simulink model "rayTrace_th"  (R2018b)
settings: Solver=VariableStepAuto  StartTime=0.0  StopTime=0  RelTol=1e-3
libraries: rayTrace_ul x4
settings Model: Creator=asiddiq2  LastModifiedBy=asiddiq2

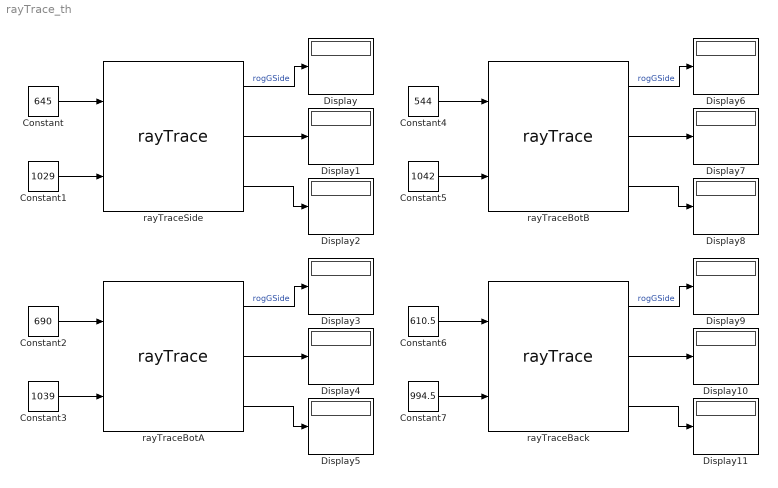
== system rayTrace_th ==
  Constant : Constant  Value=645
  Constant1 : Constant  Value=1029
  Constant2 : Constant  Value=690
  Constant3 : Constant  Value=1039
  Constant4 : Constant  Value=544
  Constant5 : Constant  Value=1042
  Constant6 : Constant  Value=610.5
  Constant7 : Constant  Value=994.5
  Display{,1..11} (12 alike) : Display
  rayTraceBack : rayTrace_ul/rayTrace  camPosVec_cm=params.prscpeCamPosVec_cm.Value  camEulAngles_deg=params.prscpeCamEulAng_deg.Value  dist2Glass_cm=params.prscpeDistancetoGlass_cm.Value  indOfRefVec=params.indexOfRefractionAGW.Value  glassPlane=3  glassThickness_cm=(3/16)*2.54  imageDimsVec_px=params.sideImageSize_px.Value  camFOV_deg=params.cameraFOV_deg.Value  Periscope=0
  rayTraceBotA : rayTrace_ul/rayTrace  camPosVec_cm=params.botCamPosVec_cm.Value  camEulAngles_deg=params.botCamEulAng_deg.Value  dist2Glass_cm=params.botDistancetoGlass_cm.Value  indOfRefVec=params.indexOfRefractionAGW.Value  glassPlane=1  glassThickness_cm=params.glassThickness_cm.Value  imageDimsVec_px=params.sideImageSize_px.Value  camFOV_deg=params.cameraFOV_deg.Value  Periscope=0
  rayTraceBotB : rayTrace_ul/rayTrace  camPosVec_cm=params.botCamPosVec_cm.Value  camEulAngles_deg=params.botCamEulAng_deg.Value  dist2Glass_cm=params.botDistancetoGlass_cm.Value  indOfRefVec=params.indexOfRefractionAGW.Value  glassPlane=1  glassThickness_cm=params.glassThickness_cm.Value  imageDimsVec_px=params.sideImageSize_px.Value  camFOV_deg=params.cameraFOV_deg.Value  Periscope=0
  rayTraceSide : rayTrace_ul/rayTrace  camPosVec_cm=params.sideCamPosVec_cm.Value  camEulAngles_deg=params.sideCamEulAng_deg.Value  dist2Glass_cm=params.sideDistancetoGlass_cm.Value  indOfRefVec=params.indexOfRefractionAGW.Value  glassPlane=2  glassThickness_cm=params.glassThickness_cm.Value  imageDimsVec_px=params.sideImageSize_px.Value  camFOV_deg=params.cameraFOV_deg.Value  Periscope=0
  wires:
  Constant/1 -> rayTraceSide/1
  Constant1/1 -> rayTraceSide/2
  rayTraceSide/2 -> Display1/1
  rayTraceSide/1 -> Display/1  "rogGSide"
  rayTraceSide/3 -> Display2/1
  rayTraceBotA/2 -> Display4/1
  rayTraceBotA/3 -> Display5/1
  rayTraceBotA/1 -> Display3/1  "rogGSide"
  rayTraceBotB/2 -> Display7/1
  rayTraceBotB/3 -> Display8/1
  rayTraceBotB/1 -> Display6/1  "rogGSide"
  rayTraceBack/2 -> Display10/1
  rayTraceBack/3 -> Display11/1
  rayTraceBack/1 -> Display9/1  "rogGSide"
  Constant3/1 -> rayTraceBotA/2
  Constant2/1 -> rayTraceBotA/1
  Constant5/1 -> rayTraceBotB/2
  Constant4/1 -> rayTraceBotB/1
  Constant7/1 -> rayTraceBack/2
  Constant6/1 -> rayTraceBack/1
